simulink model "servoInertia_sanityCheck"  (R2024b)
settings: Solver=VariableStepAuto  StartTime=0.0  StopTime=10.0  MaxStep=1e-4  RelTol=1e-3
model workspace (MATLAB code in the model file):
  | %% General Parameters
  | 
  | g = 9.81; % [m/sec^2] assuming we are on earth :)
  | 
  | %% Chosen Parameters
  | 
  | % Gearbox Ratios
  | iA = 1;
  | iBE = 1;
  | iBD = 1;
  | iG = 1;
  | iH = 1;
  | iI = 1;
  | 
  | %% Parameters from Project Description
  | 
  | % Servomotor Inertia for all joints
  | J_sm = 0.22; % [kg*m^2]
  | 
  | % Max Servomotor Current for all joints
  | Imax = 16; % [A]
  | 
  | % Motion Limits
  | thetaBE_max =  80; % [degrees]
  | thetaBE_min = -80; % [degrees]
  | thetaHI_max =  90; % [degrees]
  | thetaHI_min = -90; % [degrees]
  | 
  | % Spring Params
  | L0 = 0.750; % [m]
  | k = 100e3; % [N/m]
  | 
  | % Load Case
  | LCtolerance = 0.2; % [degrees]
  | 
  | %% Body Data from Appendix A
  | 
  | % Mass
  | mABC     = 750; % [kg]
  | mBE      = 250; % [kg]
  | mBDstick = 150; % [kg]
  | mBDblock = 500; % [kg]
  | mDF      = 50;  % [kg]
  | mEFG     = 150; % [kg]
  | mGH      = 200; % [kg]
  | mHI      = 100; % [kg]
  | mIJ      = 50;  % [kg]
  | 
  | % Mass Moment of Inertia about X-axis
  | Ix_ABC     = 50;  % [kg*m^2]
  | Ix_BE      = 1;   % [kg*m^2]
  | Ix_BDstick = 0.5; % [kg*m^2]
  | Ix_BDblock = 10;  % [kg*m^2]
  | Ix_DF      = 0.2; % [kg*m^2]
  | Ix_EFG     = 2;   % [kg*m^2]
  | Ix_GH      = 1;   % [kg*m^2]
  | Ix_HI      = 0.5; % [kg*m^2]
  | Ix_IJ      = 1;   % [kg*m^2]
  | 
  | % Mass Moment of Inertia about Y-axis
  | Iy_ABC     = 50; % [kg*m^2]
  | Iy_BE      = 20; % [kg*m^2]
  | Iy_BDstick = 8;  % [kg*m^2]
  | Iy_BDblock = 10; % [kg*m^2]
  | Iy_DF      = 1;  % [kg*m^2]
  | Iy_EFG     = 3;  % [kg*m^2]
  | Iy_GH      = 18; % [kg*m^2]
  | Iy_HI      = 2;  % [kg*m^2]
  | Iy_IJ      = 1;  % [kg*m^2]
  | 
  | % Mass Moment of Inertia about Z-axis
  | Iz_ABC     = 50; % [kg*m^2]
  | Iz_BE      = 20; % [kg*m^2]
  | Iz_BDstick = 8;  % [kg*m^2]
  | Iz_BDblock = 10; % [kg*m^2]
  | Iz_DF      = 1;  % [kg*m^2]
  | Iz_EFG     = 2;  % [kg*m^2]
  | Iz_GH      = 18; % [kg*m^2]
  | Iz_HI      = 2;  % [kg*m^2]
  | Iz_IJ      = 1;  % [kg*m^2]
  | 
  | %% Constant point distances
  | 
  | % Torquoise Block
  | EG = 0.225; % [m]
  | 
  | % End Effector
  | IJ_z = 0.248; % [m]
  | IJ_x = 0.235; % [m]
  | 
  | 
  | %% Geometry of Bodies
  | 
  | % All parameters which are not given
  | % are estimated from the figure
  | 
  | % Body AB - Blue Base
  | ABblock_L = 1; % [m]
  | ABblock_w = 4; % [m]
  | % Body BC - Blue Base Stick
  | BC_L = 0.300;  % [m]
  | BC_w = BC_L/4; % [m] NOT GIVEN, base for all sticks
  | 
  | % Body BE - Red Stick
  | BE_L = 1.050; % [m]
  | BE_w = BC_w*1.2;  % [m] NOT GIVEN
  | 
  | % Body BD - Green Block
  | BDblock_L = 0.300; % [m]
  | BDblock_w = BDblock_L; % [m] NOT GIVEN
  | % Body BD - Green Stick
  | BDstick_L = 0.800; % [m]
  | BDstick_w = BC_w;  % [m]
  | 
  | BD = 0.400; % [m]
  | 
  | % Body DF - White Stick
  | DF_L = 1.050; % [m]
  | DF_w = BC_w;  % [m]
  | 
  | % Body EFG - Torquoise block
  | EFG_L = 0.400;         % [m]
  | EFG_w = (3.5/6)*EFG_L; % [m] NOT GIVEN
  | 
  | % Body GH - Gray Stick
  | GH_L = 1.175; % [m]
  | GH_w = BC_w;  % [m] NOT GIVEN
  | 
  | % Body HI - Black Stick
  | HI_L = 0.200; % [m]
  | HI_w = BC_w;  % [m] NOT GIVEN
  | 
  | % Body IJ - (Sky Blue) End Effector Block
  | IJblock_L = (5/3.5)*IJ_x; % [m] NOT GIVEN
  | IJblock_w = (4.2/5.6)*IJ_z; % [m] NOT GIVEN
  | 
  | %% Open Loop Kinematic Parameters
  | 
  | L1 = 0.240; % [m]
  | L2 = 0.800; % [m]
  | L3 = 1.050; % [m]
  | L4 = 1.175; % [m]
  | L5 = 0.225; % [m]
  | L6 = 0.200; % [m]
  | L7 = 0.235; % [m]
  | L8 = 0.248; % [m]
  | 
  | %% Joint Visualization
  | 
  | mJ = 0.0001; % [kg]
  | 
  | % For Arms
  | r_bRJ = 0.6*BC_w; % [m]
  | l_bRJ = 2.5*BC_w; % [m]
  | r_wRJ = 0.5*BC_w; % [m]
  | l_wRJ = 2.8*BC_w; % [m]
  | 
  | % For Base
  | rB_bRJ = r_bRJ;  % [m]
  | lB_bRJ = 1.01*(ABblock_w+2*BDstick_w); % [m]
  | rB_wRJ = r_wRJ;  % [m]
  | lB_wRJ = 1.05*(ABblock_w+2*BDstick_w); % [m]
  | rBb_bRJ = r_bRJ;  % [m]
  | lBb_bRJ = 0.05*ABblock_w; % [m]
  | rBb_wRJ = r_wRJ;  % [m]
  | lBb_wRJ = 0.10*ABblock_w; % [m]
  | 
  | % r_SJ = 0.8 * w; % [m]
  | 
  | %% Point Visualization
  | 
  | P_r = 0.01; % [m]
  | 
  | %% Spring Visualization
  | 
  | spring_r = 0.05; % [m]
  | spring_L = 0.2; % [m]
  | 
  | %% Tolerances
  | 
  | maxEndEffectorAngle = 0.2; % [degrees]
undefined symbols (not defined in the file or in its folder): X, Y, Z
libraries: sm_lib x12, nesl_utility x5
settings Model: Creator=Thoma  LastModifiedBy=Thoma

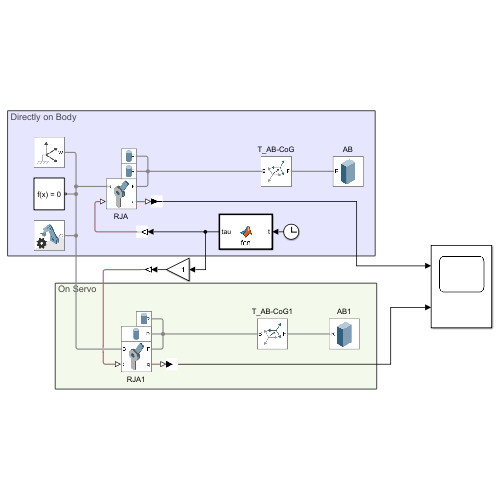
[thumbnail: Simulink's stored preview of the top-level diagram]
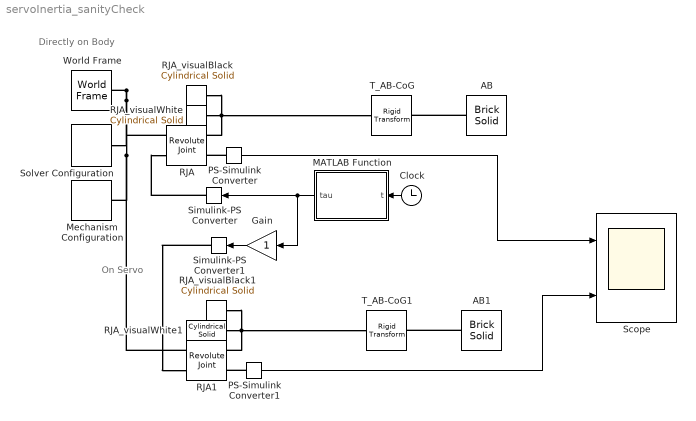
== system servoInertia_sanityCheck ==
  note: On Servo
  note: Directly on Body
  AB : sm_lib/Body Elements/Brick Solid  BrickDimensions=[ABblock_w ABblock_w ABblock_L]  BrickDimensionsUnits=m  ExportEntireGeometry=off  InertiaType=Custom  BasedOnType=Density  Density=1000  DensityUnits=kg/m^3  Mass=mABC  MassUnits=kg  CenterOfMass=[0 0 0]  CenterOfMassUnits=m  MomentsOfInertia=[Ix_ABC Iy_ABC (Iz_ABC+iA^2*J_sm)]  MomentsOfInertiaUnits=kg*m^2  ProductsOfInertia=[0 0 0]  ProductsOfInertiaUnits=kg*m^2  GraphicType=FromGeometry  MarkerShape=Sphere  MarkerSize=10  GraphicVisPropType=SimpleVisualProperties  GraphicDiffuseColor=[0 0.4471 0.7412]  GraphicOpacity=1  GraphicSpecularColor=[0.5 0.5 0.5 1.0]  GraphicAmbientColor=[0.15 0.15 0.15 1.0]  GraphicEmissiveColor=[0.0 0.0 0.0 1.0]  GraphicShininess=75  DoExposeReferenceFrame=on  SerializedFrames=<Frames/>
  AB1 : sm_lib/Body Elements/Brick Solid  BrickDimensions=[ABblock_w ABblock_w ABblock_L]  BrickDimensionsUnits=m  ExportEntireGeometry=off  InertiaType=Custom  BasedOnType=Density  Density=1000  DensityUnits=kg/m^3  Mass=mABC  MassUnits=kg  CenterOfMass=[0 0 0]  CenterOfMassUnits=m  MomentsOfInertia=[Ix_ABC Iy_ABC Iz_ABC]  MomentsOfInertiaUnits=kg*m^2  ProductsOfInertia=[0 0 0]  ProductsOfInertiaUnits=kg*m^2  GraphicType=FromGeometry  MarkerShape=Sphere  MarkerSize=10  GraphicVisPropType=SimpleVisualProperties  GraphicDiffuseColor=[0.3922 0.8314 0.07451]  GraphicOpacity=1  GraphicSpecularColor=[0.5 0.5 0.5 1.0]  GraphicAmbientColor=[0.15 0.15 0.15 1.0]  GraphicEmissiveColor=[0.0 0.0 0.0 1.0]  GraphicShininess=75  DoExposeReferenceFrame=on  SerializedFrames=<Frames/>
  Clock : Clock
  Gain : Gain
  MATLAB Function : MATLAB Function  TreatAsAtomicUnit=on
  Mechanism Configuration : sm_lib/Utilities/Mechanism Configuration  UniformGravity=Constant  GravityVector=[0 0 -g]  GravityVectorUnits=m/s^2  LinearizationDelta=0.001  JointModeTransitionNonlinearIterations=2
  PS-Simulink Converter : nesl_utility/PS-Simulink Converter  PhysicalDomain=network_engine_domain  SubClassName=ps_output  LeftPortType=input  RightPortType=output  PseudoPeriodic=off  Frequencies=[]  VectorFormat=inherit  Unit=inherit  AffineConversion=off
  PS-Simulink Converter1 : nesl_utility/PS-Simulink Converter  PhysicalDomain=network_engine_domain  SubClassName=ps_output  LeftPortType=input  RightPortType=output  PseudoPeriodic=off  Frequencies=[]  VectorFormat=inherit  Unit=inherit  AffineConversion=off
  RJA : sm_lib/Joints/Revolute Joint  JointMode=Normal  CompositeWrenchDir=FollowerOnBase  CompositeWrenchFrame=BaseFrame  SenseConstraintForce=off  SenseConstraintTorque=off  SenseTotalForce=off  SenseTotalTorque=off  PositionTargetSpecify=off  PositionTargetPriority=High  PositionTargetValue=0  PositionTargetValueUnits=deg  VelocityTargetSpecify=off  VelocityTargetPriority=High  VelocityTargetValue=0  VelocityTargetValueUnits=deg/s  EquilibriumPosition=0  EquilibriumPositionUnits=deg  SpringStiffness=0  SpringStiffnessUnits=N*m/deg  DampingCoefficient=0  DampingCoefficientUnits=N*m/(deg/s)  LowerLimitSpecify=off  LowerLimitBound=-90  LowerLimitBoundUnits=deg  LowerLimitStiffness=1e4  LowerLimitStiffnessUnits=N*m/deg  LowerLimitDamping=10  LowerLimitDampingUnits=N*m/(deg/s)  LowerLimitTransitionRegionWidth=0.1  LowerLimitTransitionRegionWidthUnits=deg  UpperLimitSpecify=off  UpperLimitBound=90  UpperLimitBoundUnits=deg  UpperLimitStiffness=1e4  UpperLimitStiffnessUnits=N*m/deg  UpperLimitDamping=10  UpperLimitDampingUnits=N*m/(deg/s)  UpperLimitTransitionRegionWidth=0.1  UpperLimitTransitionRegionWidthUnits=deg  TorqueActuationMode=InputTorque  MotionActuationMode=ComputedMotion  SensePosition=on  SenseVelocity=off  SenseAcceleration=off  SenseTorqueForce=off  SenseLowerLimitTorqueForce=off  SenseUpperLimitTorqueForce=off
  RJA1 : sm_lib/Joints/Revolute Joint  JointMode=Normal  CompositeWrenchDir=FollowerOnBase  CompositeWrenchFrame=BaseFrame  SenseConstraintForce=off  SenseConstraintTorque=off  SenseTotalForce=off  SenseTotalTorque=off  PositionTargetSpecify=off  PositionTargetPriority=High  PositionTargetValue=0  PositionTargetValueUnits=deg  VelocityTargetSpecify=off  VelocityTargetPriority=High  VelocityTargetValue=0  VelocityTargetValueUnits=deg/s  EquilibriumPosition=0  EquilibriumPositionUnits=deg  SpringStiffness=0  SpringStiffnessUnits=N*m/deg  DampingCoefficient=0  DampingCoefficientUnits=N*m/(deg/s)  LowerLimitSpecify=off  LowerLimitBound=-90  LowerLimitBoundUnits=deg  LowerLimitStiffness=1e4  LowerLimitStiffnessUnits=N*m/deg  LowerLimitDamping=10  LowerLimitDampingUnits=N*m/(deg/s)  LowerLimitTransitionRegionWidth=0.1  LowerLimitTransitionRegionWidthUnits=deg  UpperLimitSpecify=off  UpperLimitBound=90  UpperLimitBoundUnits=deg  UpperLimitStiffness=1e4  UpperLimitStiffnessUnits=N*m/deg  UpperLimitDamping=10  UpperLimitDampingUnits=N*m/(deg/s)  UpperLimitTransitionRegionWidth=0.1  UpperLimitTransitionRegionWidthUnits=deg  TorqueActuationMode=InputTorque  MotionActuationMode=ComputedMotion  SensePosition=on  SenseVelocity=off  SenseAcceleration=off  SenseTorqueForce=off  SenseLowerLimitTorqueForce=off  SenseUpperLimitTorqueForce=off
  RJA_visualBlack : sm_lib/Body Elements/Cylindrical Solid  CylinderRadius=rBb_bRJ  CylinderRadiusUnits=m  CylinderLength=lBb_bRJ  CylinderLengthUnits=m  ExportEntireGeometry=off  InertiaType=CalculateFromGeometry  BasedOnType=Mass  Density=1000  DensityUnits=kg/m^3  Mass=mJ  MassUnits=kg  CenterOfMass=[0 0 0]  CenterOfMassUnits=m  MomentsOfInertia=[1 1 1]  MomentsOfInertiaUnits=kg*m^2  ProductsOfInertia=[0 0 0]  ProductsOfInertiaUnits=kg*m^2  GraphicType=FromGeometry  MarkerShape=Sphere  MarkerSize=10  GraphicVisPropType=AdvancedVisualProperties  GraphicDiffuseColor=[0.0 0.0 0.0]  GraphicOpacity=1.0  GraphicSpecularColor=[0.5 0.5 0.5 1.0]  GraphicAmbientColor=[0.15 0.15 0.15 1.0]  GraphicEmissiveColor=[0.0 0.0 0.0 1.0]  GraphicShininess=75  DoExposeReferenceFrame=on  SerializedFrames=<Frames/>
  RJA_visualBlack1 : sm_lib/Body Elements/Cylindrical Solid  CylinderRadius=rBb_bRJ  CylinderRadiusUnits=m  CylinderLength=lBb_bRJ  CylinderLengthUnits=m  ExportEntireGeometry=off  InertiaType=CalculateFromGeometry  BasedOnType=Mass  Density=1000  DensityUnits=kg/m^3  Mass=mJ  MassUnits=kg  CenterOfMass=[0 0 0]  CenterOfMassUnits=m  MomentsOfInertia=[1 1 1]  MomentsOfInertiaUnits=kg*m^2  ProductsOfInertia=[0 0 0]  ProductsOfInertiaUnits=kg*m^2  GraphicType=FromGeometry  MarkerShape=Sphere  MarkerSize=10  GraphicVisPropType=AdvancedVisualProperties  GraphicDiffuseColor=[0.0 0.0 0.0]  GraphicOpacity=1.0  GraphicSpecularColor=[0.5 0.5 0.5 1.0]  GraphicAmbientColor=[0.15 0.15 0.15 1.0]  GraphicEmissiveColor=[0.0 0.0 0.0 1.0]  GraphicShininess=75  DoExposeReferenceFrame=on  SerializedFrames=<Frames/>
  RJA_visualWhite : sm_lib/Body Elements/Cylindrical Solid  CylinderRadius=rBb_wRJ  CylinderRadiusUnits=m  CylinderLength=lBb_wRJ  CylinderLengthUnits=m  ExportEntireGeometry=off  InertiaType=CalculateFromGeometry  BasedOnType=Mass  Density=1000  DensityUnits=kg/m^3  Mass=mJ  MassUnits=kg  CenterOfMass=[0 0 0]  CenterOfMassUnits=m  MomentsOfInertia=[1 1 J_sm*iA^2]  MomentsOfInertiaUnits=kg*m^2  ProductsOfInertia=[0 0 0]  ProductsOfInertiaUnits=kg*m^2  GraphicType=FromGeometry  MarkerShape=Sphere  MarkerSize=10  GraphicVisPropType=SimpleVisualProperties  GraphicDiffuseColor=[1.0 1.0 1.0]  GraphicOpacity=1.0  GraphicSpecularColor=[0.5 0.5 0.5 1.0]  GraphicAmbientColor=[0.15 0.15 0.15 1.0]  GraphicEmissiveColor=[0.0 0.0 0.0 1.0]  GraphicShininess=75  DoExposeReferenceFrame=on  SerializedFrames=<Frames/>
  RJA_visualWhite1 : sm_lib/Body Elements/Cylindrical Solid  CylinderRadius=rBb_wRJ  CylinderRadiusUnits=m  CylinderLength=lBb_wRJ  CylinderLengthUnits=m  ExportEntireGeometry=off  InertiaType=Custom  BasedOnType=Mass  Density=1000  DensityUnits=kg/m^3  Mass=mJ  MassUnits=kg  CenterOfMass=[0 0 0]  CenterOfMassUnits=m  MomentsOfInertia=[1 1 J_sm*iA^2]  MomentsOfInertiaUnits=kg*m^2  ProductsOfInertia=[0 0 0]  ProductsOfInertiaUnits=kg*m^2  GraphicType=FromGeometry  MarkerShape=Sphere  MarkerSize=10  GraphicVisPropType=SimpleVisualProperties  GraphicDiffuseColor=[1.0 1.0 1.0]  GraphicOpacity=1.0  GraphicSpecularColor=[0.5 0.5 0.5 1.0]  GraphicAmbientColor=[0.15 0.15 0.15 1.0]  GraphicEmissiveColor=[0.0 0.0 0.0 1.0]  GraphicShininess=75  DoExposeReferenceFrame=on  SerializedFrames=<Frames/>
  Scope : Scope  NumInputPorts=2
  Simulink-PS Converter : nesl_utility/Simulink-PS Converter  PhysicalDomain=network_engine_domain  SubClassName=ps_input  LeftPortType=input  RightPortType=output  PseudoPeriodic=off  Frequencies=[]  NoiseDistribution=none  NoiseParameters=[]  Unit=1  AffineConversion=off  FilteringAndDerivatives=provide  SimscapeFilterOrder=1  InputFilterTimeConstant=0.001  UdotUserProvided=0
  Simulink-PS Converter1 : nesl_utility/Simulink-PS Converter  PhysicalDomain=network_engine_domain  SubClassName=ps_input  LeftPortType=input  RightPortType=output  PseudoPeriodic=off  Frequencies=[]  NoiseDistribution=none  NoiseParameters=[]  Unit=1  AffineConversion=off  FilteringAndDerivatives=provide  SimscapeFilterOrder=1  InputFilterTimeConstant=0.001  UdotUserProvided=0
  Solver Configuration : nesl_utility/Solver Configuration  PhysicalDomain=network_engine_domain  SubClassName=solver  LeftPortType=input  RightPortType=generic  Tones=[]  Harmonics=[]  SimulateNoise=off  Profile=off  UseLocalSampling=off  EnableSwitchedLinearOptims=on  FrequencyDomain=off  UseCCode=off  RelTol=0.001  AbsTol=1e-06  MinStep=1e-09  ToWorkspace=off  RevertToSquareIcSolve=off  NumHomotopyIterations=100  PhasorMode=off  PhasorModeNumHarmonics=1  ConsistencySolver=NEWTON_FTOL  IndexReductionMethod=DerivativeReplacement  DoDC=off  ResidualTolerance=1e-9  ConsistencyTolSource=GLOBAL  ConsistencyAbsTol=0.001  ConsistencyRelTol=0.001  ConsistencyTolFactor=0.001  UseLocalSolver=off  LocalSolverChoice=NE_BACKWARD_EULER_ADVANCER  ResolveIndetEquations=on  FunctionEvalNumThread=1  LocalSolverSampleTime=.001  DoFixedCost=off  MaxNonlinIter=3  MaxModeIter=2  ComputeImpulses=off  ImpulseIterations=2  LinearAlgebra=Sparse  LinearAlgebraNumThread=0  EquationFormulation=NE_TIME_EF  DelaysMemoryBudget=1024  AutomaticFiltering=on  FilteringTimeConstant=0.001  PartitionStorageMethod=AS_NEEDED  PartitionMemoryBudget=1024  PartitionMethod=FAST  MultibodyUseLocalSolver=off  MultibodyLocalSolverChoice=ODE1  MultibodyLocalSolverSampleTime=0.001
  T_AB-CoG : sm_lib/Frames and Transforms/Rigid Transform  RotationMethod=None  FollAlignAxisA=+X  BaseAlignAxisA=+Y  FollAlignAxisB=+Y  BaseAlignAxisB=+Z  RotationStandardAxis=+Z  RotationAngle=0  RotationAngleUnits=deg  RotationArbitraryAxis=[0 0 1]  RotationSequenceAxes=FollowerAxes  RotationSequence=XYX  RotationSequenceAngles=[0 0 0]  RotationSequenceAnglesUnits=deg  RotationMatrix=[1 0 0;0 1 0;0 0 1]  Quaternion=[1 0 0 0]  TranslationMethod=Cartesian  TranslationCartesianOffset=[1 0 ABblock_L/2]  TranslationCartesianOffsetUnits=m  TranslationStandardAxis=+Z  TranslationStandardOffset=0  TranslationStandardOffsetUnits=m  TranslationROffset=0  TranslationROffsetUnits=m  TranslationThetaOffset=0  TranslationThetaOffsetUnits=deg  TranslationZOffset=0  TranslationZOffsetUnits=m
  T_AB-CoG1 : sm_lib/Frames and Transforms/Rigid Transform  RotationMethod=None  FollAlignAxisA=+X  BaseAlignAxisA=+Y  FollAlignAxisB=+Y  BaseAlignAxisB=+Z  RotationStandardAxis=+Z  RotationAngle=0  RotationAngleUnits=deg  RotationArbitraryAxis=[0 0 1]  RotationSequenceAxes=FollowerAxes  RotationSequence=XYX  RotationSequenceAngles=[0 0 0]  RotationSequenceAnglesUnits=deg  RotationMatrix=[1 0 0;0 1 0;0 0 1]  Quaternion=[1 0 0 0]  TranslationMethod=Cartesian  TranslationCartesianOffset=[1 0 ABblock_L/2]  TranslationCartesianOffsetUnits=m  TranslationStandardAxis=+Z  TranslationStandardOffset=0  TranslationStandardOffsetUnits=m  TranslationROffset=0  TranslationROffsetUnits=m  TranslationThetaOffset=0  TranslationThetaOffsetUnits=deg  TranslationZOffset=0  TranslationZOffsetUnits=m
  World Frame : sm_lib/Frames and Transforms/World Frame
  wires:
  PS-Simulink Converter/1 -> Scope/1
  Clock/1 -> MATLAB Function/1(t)
  PS-Simulink Converter1/1 -> Scope/2
  MATLAB Function/1(tau) -> Gain/1, Simulink-PS Converter/1
  Gain/1 -> Simulink-PS Converter1/1
  connections:
  RJA_visualWhite/RConn1 -- RJA/RConn1 -- T_AB-CoG/LConn1 -- RJA_visualBlack/RConn1
  World Frame/RConn1 -- Solver Configuration/RConn1 -- RJA1/LConn1 -- Mechanism Configuration/RConn1 -- RJA/LConn1
  AB/RConn1 -- T_AB-CoG/RConn1
  PS-Simulink Converter/LConn1 -- RJA/RConn2
  Simulink-PS Converter/RConn1 -- RJA/LConn2
  RJA_visualWhite1/RConn1 -- RJA1/RConn1 -- T_AB-CoG1/LConn1 -- RJA_visualBlack1/RConn1
  PS-Simulink Converter1/LConn1 -- RJA1/RConn2
  AB1/RConn1 -- T_AB-CoG1/RConn1
  Simulink-PS Converter1/RConn1 -- RJA1/LConn2

== matlab function servoInertia_sanityCheck/MATLAB Function ==
  data: t input; tau output
function tau = fcn(t)

A = 800*pi;
tau = A*sin(2*pi*t);
